simulink model "modelLab2"  (R2022b)
settings: Solver=VariableStepAuto  StartTime=0.0  StopTime=1.5 * Ts  RelTol=1e-3
values from neighbouring files (symbols this model uses):
  A = [0 1 0 0; constA 0 0 (constA .* constC)./(n .* g); 0 0 0 1; 0 0 0 -constC]    [lab2.m]
  B = [0; (constA .* constD)./(n .* g); 0; constD]    [lab2.m]
  C = [1 0 0 0]    [lab2.m]
  D = zeros(1,4)    [lab2.m]
  x0 = [0.17; 0; 0; 0]    [lab2.m]
undefined symbols (not defined in the file or in its folder): Af, Bf, Cf, Df, K
libraries: simulink x1
settings Model: Creator=fwah  LastModifiedBy=fwah

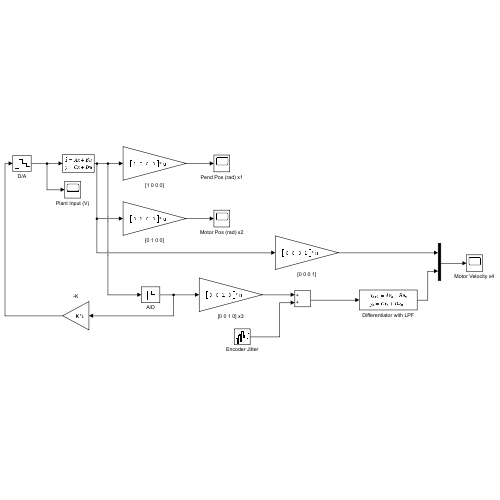
[thumbnail: Simulink's stored preview of the top-level diagram]
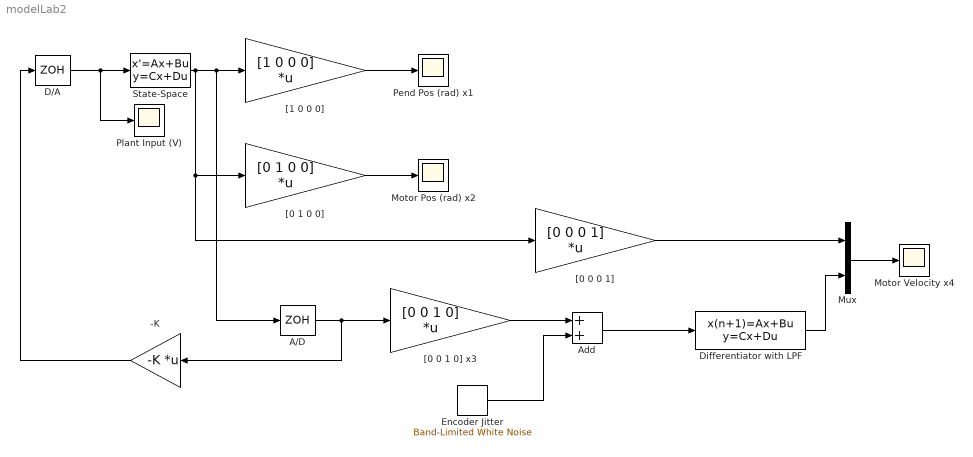
== system modelLab2 ==
  -K : Gain  Gain=-K  Multiplication=Matrix(K*u)
  A/D : ZeroOrderHold  SampleTime=-1
  Add : Sum
  D/A : ZeroOrderHold  SampleTime=-1
  Differentiator with LPF : DiscreteStateSpace  A=Af  B=Bf  C=Cf  D=Df  SampleTime=-1
  Encoder Jitter : simulink/Sources/Band-Limited White Noise  Cov=[0.1]  Ts=0.1  seed=[23341]
  Motor Pos (rad) x2 : Scope
  Motor Velocity x4 : Scope
  Mux : Mux  Inputs=2
  Pend Pos (rad) x1 : Scope
  Plant Input (V) : Scope
  State-Space : StateSpace  A=A  B=B  C=C  D=D  InitialCondition=x0
  "[0 0 0 1]" : Gain  Gain=[0 0 0 1]  Multiplication=Matrix(K*u)
  "[0 0 1 0] x3" : Gain  Gain=[0 0 1 0]  Multiplication=Matrix(K*u)
  "[0 1 0 0]" : Gain  Gain=[0 1 0 0]  Multiplication=Matrix(K*u)
  "[1 0 0 0]" : Gain  Gain=[1 0 0 0]  Multiplication=Matrix(K*u)
  wires:
  Differentiator with LPF/1 -> Mux/2
  D/A/1 -> State-Space/1, Plant Input (V)/1
  -K/1 -> D/A/1
  "[0 1 0 0]"/1 -> Motor Pos (rad) x2/1
  Mux/1 -> Motor Velocity x4/1
  State-Space/1 -> "[0 1 0 0]"/1, "[0 0 0 1]"/1, A/D/1, "[1 0 0 0]"/1
  Add/1 -> Differentiator with LPF/1
  "[0 0 0 1]"/1 -> Mux/1
  "[1 0 0 0]"/1 -> Pend Pos (rad) x1/1
  A/D/1 -> -K/1, "[0 0 1 0] x3"/1
  "[0 0 1 0] x3"/1 -> Add/1
  Encoder Jitter/1 -> Add/2
